simulink model "F4_CAN_Networking"  (R2018b)
settings: Solver=FixedStepAuto  StartTime=0.0  StopTime=10.0  FixedStep=0.25  RelTol=1e-3
undefined symbols (not defined in the file): CAN_MESSAGE
libraries: GPIO_Lib x9, CAN_Lib x7, STM32_Config_Lib x1, canmsglib x1
settings Model: Creator=reynaudp  LastModifiedBy=fenard1
settings SolverCC: InsertRTBMode=Always
settings DataIOCC: LimitDataPoints=on  SaveFormat=Array  ReturnWorkspaceOutputs=on
settings OptimizationCC: DefaultParameterBehavior=Inlined  DefaultUnderspecifiedDataType=single  InlineInvariantSignals=on  PassReuseOutputArgsAs=Individual arguments  LifeSpan=1
settings DebuggingCC: ReadBeforeWriteMsg=DisableAll  WriteAfterWriteMsg=DisableAll  WriteAfterReadMsg=DisableAll  SolverPrmCheckMsg=warning  MultiTaskDSMMsg=none  AllowSymbolicDim=off  StrictBusMsg=WarnOnBusTreatedAsVector  SFUnexpectedBacktrackingDiag=warning  SFNoUnconditionalDefaultTransitionDiag=warning  SFUndirectedBroadcastEventsDiag=error  SFExecutionAtInitializationDiag=none
settings HardwareCC: ProdBitPerPointer=32  ProdBitPerSizeT=32  ProdBitPerPtrDiffT=32  ProdLargestAtomicInteger=Integer  ProdWordSize=32  ProdHWDeviceType=STMicroelectronics->STM32 32-bit Cortex-M
settings ModelReferenceCC: UpdateModelReferenceTargets=IfOutOfDate  PropagateSignalLabelsOutOfModel=off
settings SFSimCC: SFSimEcho=off  SimUseLocalCustomCode=off  CompileTimeRecursionLimit=0  EnableRuntimeRecursion=off  MATLABDynamicMemAlloc=off
settings RTWCC: SystemTargetFile=stm32.tlc  TemplateMakefile=stm32.tmf  Description=stm32 (Embedded Target)  GenerateReport=on  RTWVerbose=off  RTWUseLocalCustomCode=off  Toolchain=Microsoft Windows SDK v7.1 | nmake (64-bit Windows)  IncludeHyperlinkInReport=on
settings CodeAppCC: IgnoreCustomStorageClasses=off  CustomSymbolStrType=$N$R$M  SimulinkBlockComments=off
settings STFCustomTargetCC: CodeReplacementLibrary=ARM CMSIS SIN COS  ParMdlRefBuildCompliant=on  IncludeMdlTerminateFcn=off  CombineOutputUpdateFcns=on  ERTCustomFileBanners=on  SupportContinuousTime=off  SupportNonInlinedSFcns=off  RemoveResetFunc=on  ParenthesesLevel=Maximum  CastingMode=Standards  MATLABClassNameForMDSCustomization=Simulink.SoftwareTarget.ERTCustomization  SystemTargetFile=stm32.tlc
settings ERTTargetCC: CodeReplacementLibrary=ARM CMSIS SIN COS  MultiwordLength=2048  CompOptLevelCompliant=off  ConcurrentExecutionCompliant=off  IncludeMdlTerminateFcn=off  ParenthesesLevel=Maximum  CastingMode=Standards  ModelStepFunctionPrototypeControlCompliant=off  CPPClassGenCompliant=off  UseToolchainInfoCompliant=off  ERTSrcFileBannerTemplate=sourceFileTemplate.cgt  ERTHdrFileBannerTemplate=sourceFileTemplate.cgt  ERTDataSrcFileTemplate=sourceFileTemplate.cgt  ERTDataHdrFileTemplate=sourceFileTemplate.cgt  ERTCustomFileTemplate=customRoutineProcess.tlc  ConvertIfToSwitch=off  SuppressUnreachableDefaultCases=off  EnableSignedLeftShifts=off  EnableSignedRightShifts=off
settings ConfigComp: CovMetricSettings=dw  CovHtmlReporting=on  CovSaveCumulativeToWorkspaceVar=on  CovSaveSingleToWorkspaceVar=on  CovExternalEMLEnable=off  CovSFcnEnable=off

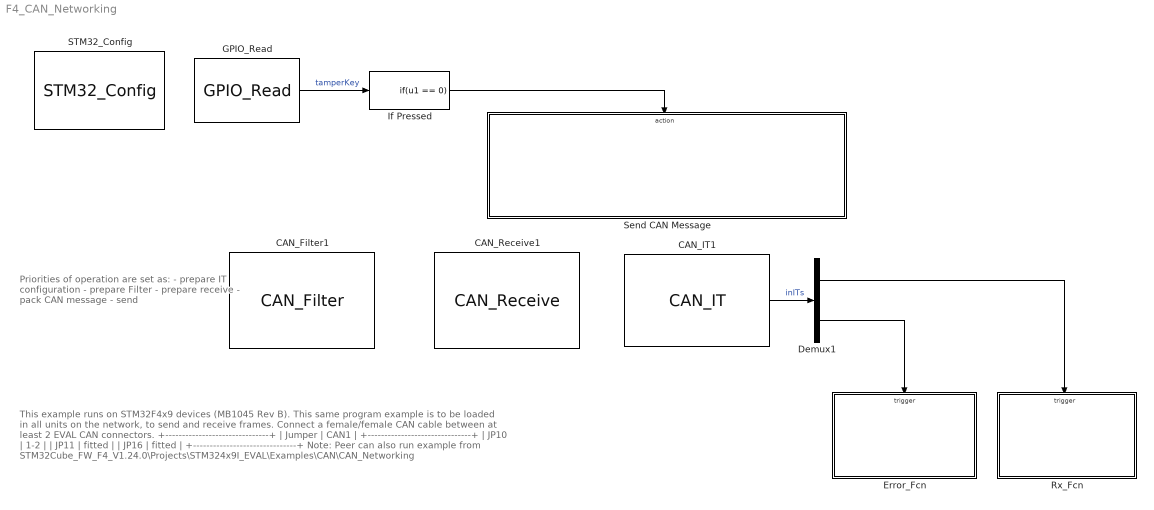
== system F4_CAN_Networking ==
  note: This example runs on STM32F4x9 devices (MB1045 Rev B).
      |
      | This same program example is to be loaded in all units on the network, to send and receive frames.
      |
      | Connect a female/female CAN cable between at least 2 EVAL CAN connectors.
      |
      | +-------------------------------+
      | | Jumper | CAN1 |
      | +-------------------------------+
      | | JP10 | 1-2 |
      | | JP11 | fitted |
      | | JP16 | fitted |
      | +-------------------------------+
      |
      | Note: Peer can also run example from STM32Cube_FW_F4_V1.24.0\Projects\STM324x9I_EVAL\Examples\CAN\CAN_Networking
  note: Priorities of operation are set as:
      | - prepare IT configuration
      | - prepare Filter
      | - prepare receive
      |
      | - pack CAN message
      | - send
  CAN_Filter1 : CAN_Lib/CAN_Filter  Priority=2  CAN_name=CAN1  CAN_Filter_Activation=on  CAN_Filter_Scale=CAN_FILTERSCALE_32BIT  CAN_Filter_Mask_Id_High=0  CAN_Filter_Mask_Id_Low=0  CAN_Filter_Id_High=0  CAN_Filter_Id_Low=0  CAN_Filter_FIFO_Assignment=CAN_FIFO0  CAN_Filter_Bank=0  CAN_Filter_Mode=CAN_FILTERMODE_IDMASK  CAN_Filter_Slave_Start_Bank=14
      settings: AttributesFormatString=Priority=%<Priority>  SourceProductName=Target Support Package - STM32 Adapter
  CAN_IT1 : CAN_Lib/CAN_IT  Priority=1  CAN_name=CAN1  CAN_Mode=Master  CAN_It=on  CAN_RX_It=on  CAN_TX_It=off  CAN_ERROR_It=on
      settings: AttributesFormatString=Priority=%<Priority>  SourceProductName=Target Support Package - STM32 Adapter
  CAN_Receive1 : CAN_Lib/CAN_Receive  Priority=3  CAN_name=CAN1  CAN_Mode=Master  CAN_It=on  CAN_Fifo=CAN_FIFO0
      settings: AttributesFormatString=Priority=%<Priority>  SourceProductName=Target Support Package - STM32 Adapter
  Demux1 : Demux  Outputs=2
  Error_Fcn : Subsystem  TreatAsAtomicUnit=on
  GPIO_Read : GPIO_Lib/GPIO_Read  Port_name=GPIOC  Pin_0=off  Pin_1=off  Pin_2=off  Pin_3=off  Pin_4=off  Pin_5=off  Pin_6=off  Pin_7=off  Pin_8=off  Pin_9=off  Pin_10=off  Pin_11=off  Pin_12=off  Pin_13=on  Pin_14=off  Pin_15=off  PinList=GPIOC13
      settings: SourceProductName=Target Support Package - STM32 Adapter
  If Pressed : If  IfExpression=u1 == 0  ShowElse=off
  Rx_Fcn : Subsystem  TreatAsAtomicUnit=on
  STM32_Config : STM32_Config_Lib/STM32_Config  Priority=0  Project_Path=.\  Config_File=F4_CAN_Networking.ioc  MCU_Name=STM32F439NIHx
      settings: SourceProductName=Target Support Package - STM32 Adapter
  Send CAN Message : Subsystem  TreatAsAtomicUnit=on  RTWFcnName=sendMessage
      settings: RTWFcnNameOpts=User specified
  wires:
  Demux1/2 -> Error_Fcn/Trigger
  CAN_IT1/1 -> Demux1/1  "inITs"
  Demux1/1 -> Rx_Fcn/Trigger
  GPIO_Read/1 -> If Pressed/1  "tamperKey"
  If Pressed/1 -> Send CAN Message/Action

== system F4_CAN_Networking/Error_Fcn ==
  Error_Fcn : TriggerPort  TriggerType=function-call  VariantControl=Variant
  CAN_Reset : CAN_Lib/CAN_Reset  CAN_name=CAN1
      settings: SourceProductName=Target Support Package - STM32 Adapter

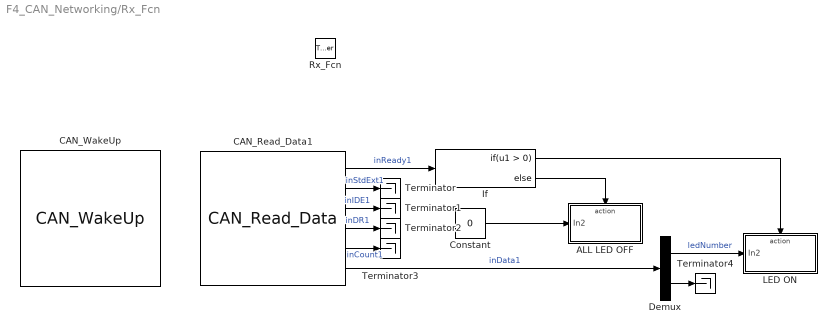
== system F4_CAN_Networking/Rx_Fcn ==
  Rx_Fcn : TriggerPort  TriggerType=function-call  VariantControl=Variant
  ALL LED OFF : Subsystem  TreatAsAtomicUnit=on
      settings: RTWSystemCode=Inline
  CAN_Read_Data1 : CAN_Lib/CAN_Read_Data  CAN_name=CAN1  CAN_Fifo=CAN_FIFO0  CAN_MsgType=off
      settings: SourceProductName=Target Support Package - STM32 Adapter
  CAN_WakeUp : CAN_Lib/CAN_WakeUp  CAN_name=CAN1  CAN_Mode=Master  CAN_It=on
      settings: SourceProductName=Target Support Package - STM32 Adapter
  Constant : Constant  Value=0  OutDataTypeStr=uint8
  Demux : Demux  Outputs=2
  If : If
  LED ON : Subsystem  TreatAsAtomicUnit=on
      settings: RTWSystemCode=Inline
  Terminator{,1..4} (5 alike) : Terminator
  wires:
  CAN_Read_Data1/6 -> Demux/1  "inData1"
  CAN_Read_Data1/1 -> If/1  "inReady1"
  If/1 -> LED ON/Action
  Demux/1 -> LED ON/1(In2)  "ledNumber"
  If/2 -> ALL LED OFF/Action
  Constant/1 -> ALL LED OFF/1(In2)
  CAN_Read_Data1/2 -> Terminator/1  "inStdExt1"
  CAN_Read_Data1/3 -> Terminator1/1  "inIDE1"
  CAN_Read_Data1/4 -> Terminator2/1  "inDR1"
  CAN_Read_Data1/5 -> Terminator3/1  "inCount1"
  Demux/2 -> Terminator4/1

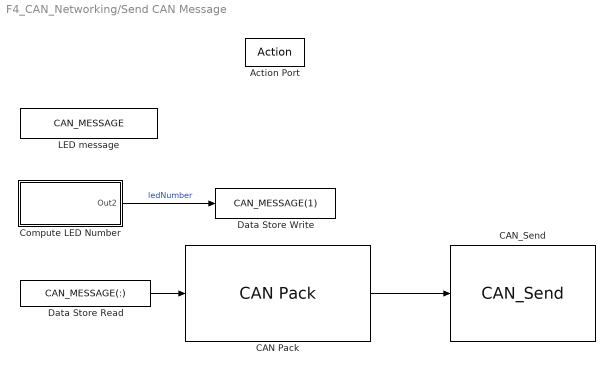
== system F4_CAN_Networking/Send CAN Message ==
  Action Port : ActionPort  ActionType=then
  CAN Pack : canmsglib/CAN Pack  Priority=22  MsgList=(none)  MsgName=CAN Msg  MsgIDType=Standard (11-bit identifier)  MsgIdentifier=801  MsgLength=2  SignalInfo=Signal1$0$8$1$1$1$0$1$0$-Inf$Inf$#  NSignals=1  StartBits=str2num('[int32(0)]')  SignalSizes=str2num('[int32(8)]')  ByteOrders=str2num('[int32(1)]')  DataTypes=str2num('[int32(1)]')  MultiplexTypes=str2num('[int32(1)]')  MultiplexValues=str2num('[double(0)]')  Factors=str2num('[double(1)]')  Offsets=str2num('[double(0)]')  Minimums=str2num('[double(-Inf)]')  Maximums=str2num('[double(Inf)]')  Remote=off  ApplyMinMax=off  BusOutput=off
      settings: AttributesFormatString=Priority=%<Priority>  SourceProductName=Simulink Real-Time  SourceProductBaseCode=XP  DataFormat=raw data
  CAN_Send : CAN_Lib/CAN_Send  Priority=23  CAN_name=CAN1  CAN_Mode=Master  CAN_It=off  CAN_MsgType=on
      settings: AttributesFormatString=Priority=%<Priority>  SourceProductName=Target Support Package - STM32 Adapter
  Compute LED Number : Subsystem  Priority=21  TreatAsAtomicUnit=on  RTWFcnName=computeLedNumber
      settings: AttributesFormatString=Priority=%<Priority>  RTWFcnNameOpts=User specified
  Data Store Read : DataStoreRead  DataStoreName=CAN_MESSAGE  DataStoreElements=CAN_MESSAGE(:)
  Data Store Write : DataStoreWrite  DataStoreName=CAN_MESSAGE  DataStoreElements=CAN_MESSAGE(1)
  LED message : DataStoreMemory  DataStoreName=CAN_MESSAGE  ReadBeforeWriteMsg=warning  WriteAfterWriteMsg=warning  WriteAfterReadMsg=warning  InitialValue=[1, 173]  ShowAdditionalParam=off  OutDataTypeStr=uint8
  wires:
  Compute LED Number/1(Out2) -> Data Store Write/1  "ledNumber"
  CAN Pack/1 -> CAN_Send/1
  Data Store Read/1 -> CAN Pack/1

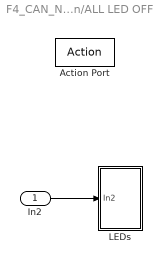
== system F4_CAN_Networking/Rx_Fcn/ALL LED OFF ==
  In2 : Inport  OutDataTypeStr=uint8
  Action Port : ActionPort  ActionType=else
  LEDs : Subsystem
  wires:
  In2/1 -> LEDs/1(In2)

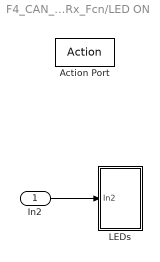
== system F4_CAN_Networking/Rx_Fcn/LED ON ==
  In2 : Inport  OutDataTypeStr=uint8
  Action Port : ActionPort  ActionType=then
  LEDs : Subsystem  TreatAsAtomicUnit=on  RTWFcnName=setLed
      settings: RTWFcnNameOpts=User specified
  wires:
  In2/1 -> LEDs/1(In2)

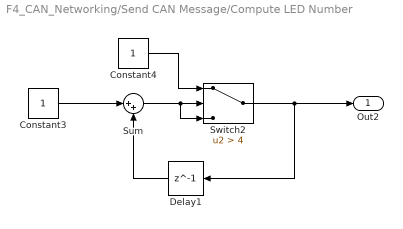
== system F4_CAN_Networking/Send CAN Message/Compute LED Number ==
  Constant3 : Constant  OutDataTypeStr=uint8
  Constant4 : Constant  OutDataTypeStr=uint8
  Delay1 : Delay  DelayLength=1  InitialCondition=0
  Sum : Sum  Inputs=|++
  Switch2 : Switch  Criteria=u2 > Threshold  Threshold=4  OutDataTypeStr=uint8
  Out2 : Outport
  wires:
  Sum/1 -> Switch2/3, Switch2/2
  Constant4/1 -> Switch2/1
  Delay1/1 -> Sum/2
  Constant3/1 -> Sum/1
  Switch2/1 -> Delay1/1, Out2/1

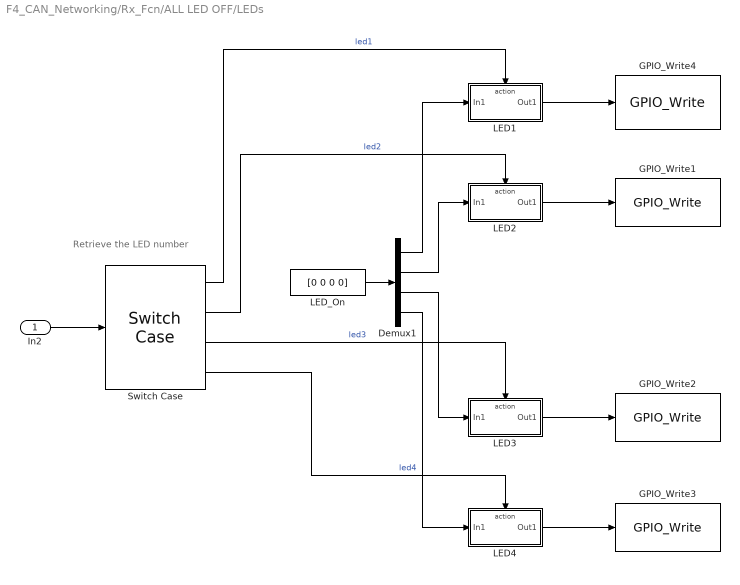
== system F4_CAN_Networking/Rx_Fcn/ALL LED OFF/LEDs ==
  note: Retrieve the LED number
  In2 : Inport  OutDataTypeStr=uint8
  Demux1 : Demux
  GPIO_Write1 : GPIO_Lib/GPIO_Write  Port_name=GPIOG  Pin0=off  Toggle_Pin0=off  Pin1=off  Toggle_Pin1=off  Pin2=off  Toggle_Pin2=off  Pin3=off  Toggle_Pin3=off  Pin4=off  Toggle_Pin4=off  Pin5=off  Toggle_Pin5=off  Pin6=off  Toggle_Pin6=off  Pin7=on  Toggle_Pin7=off  Pin8=off  Toggle_Pin8=off  Pin9=off  Toggle_Pin9=off  Pin10=off  Toggle_Pin10=off  Pin11=off  Toggle_Pin11=off  Pin12=off  Toggle_Pin12=off  Pin13=off  Toggle_Pin13=off  Pin14=off  Toggle_Pin14=off  Pin15=off  Toggle_Pin15=off  PinList="GPIOG6   7  10  12"
      settings: SourceProductName=Target Support Package - STM32 Adapter
  GPIO_Write2 : GPIO_Lib/GPIO_Write  Port_name=GPIOG  Pin0=off  Toggle_Pin0=off  Pin1=off  Toggle_Pin1=off  Pin2=off  Toggle_Pin2=off  Pin3=off  Toggle_Pin3=off  Pin4=off  Toggle_Pin4=off  Pin5=off  Toggle_Pin5=off  Pin6=off  Toggle_Pin6=off  Pin7=off  Toggle_Pin7=off  Pin8=off  Toggle_Pin8=off  Pin9=off  Toggle_Pin9=off  Pin10=on  Toggle_Pin10=off  Pin11=off  Toggle_Pin11=off  Pin12=off  Toggle_Pin12=off  Pin13=off  Toggle_Pin13=off  Pin14=off  Toggle_Pin14=off  Pin15=off  Toggle_Pin15=off  PinList="GPIOG6   7  10  12"
      settings: SourceProductName=Target Support Package - STM32 Adapter
  GPIO_Write3 : GPIO_Lib/GPIO_Write  Port_name=GPIOG  Pin0=off  Toggle_Pin0=off  Pin1=off  Toggle_Pin1=off  Pin2=off  Toggle_Pin2=off  Pin3=off  Toggle_Pin3=off  Pin4=off  Toggle_Pin4=off  Pin5=off  Toggle_Pin5=off  Pin6=off  Toggle_Pin6=off  Pin7=off  Toggle_Pin7=off  Pin8=off  Toggle_Pin8=off  Pin9=off  Toggle_Pin9=off  Pin10=off  Toggle_Pin10=off  Pin11=off  Toggle_Pin11=off  Pin12=on  Toggle_Pin12=off  Pin13=off  Toggle_Pin13=off  Pin14=off  Toggle_Pin14=off  Pin15=off  Toggle_Pin15=off  PinList="GPIOG6   7  10  12"
      settings: SourceProductName=Target Support Package - STM32 Adapter
  GPIO_Write4 : GPIO_Lib/GPIO_Write  Port_name=GPIOG  Pin0=off  Toggle_Pin0=off  Pin1=off  Toggle_Pin1=off  Pin2=off  Toggle_Pin2=off  Pin3=off  Toggle_Pin3=off  Pin4=off  Toggle_Pin4=off  Pin5=off  Toggle_Pin5=off  Pin6=on  Toggle_Pin6=off  Pin7=off  Toggle_Pin7=off  Pin8=off  Toggle_Pin8=off  Pin9=off  Toggle_Pin9=off  Pin10=off  Toggle_Pin10=off  Pin11=off  Toggle_Pin11=off  Pin12=off  Toggle_Pin12=off  Pin13=off  Toggle_Pin13=off  Pin14=off  Toggle_Pin14=off  Pin15=off  Toggle_Pin15=off  PinList="GPIOG6   7  10  12"
      settings: SourceProductName=Target Support Package - STM32 Adapter
  LED1 : Subsystem  TreatAsAtomicUnit=on
  LED2 : Subsystem  TreatAsAtomicUnit=on
  LED3 : Subsystem  TreatAsAtomicUnit=on
  LED4 : Subsystem  TreatAsAtomicUnit=on
  LED_On : Constant  Value=[0 0 0 0]  OutDataTypeStr=uint32
  Switch Case : SwitchCase  CaseConditions={1,2,3,4}  ShowDefaultCase=off
  wires:
  Demux1/2 -> LED2/1(In1)
  LED_On/1 -> Demux1/1
  Switch Case/3 -> LED3/Action  "led3"
  Demux1/3 -> LED3/1(In1)
  LED4/1(Out1) -> GPIO_Write3/1
  LED1/1(Out1) -> GPIO_Write4/1
  In2/1 -> Switch Case/1
  LED3/1(Out1) -> GPIO_Write2/1
  Switch Case/4 -> LED4/Action  "led4"
  Demux1/4 -> LED4/1(In1)
  LED2/1(Out1) -> GPIO_Write1/1
  Switch Case/1 -> LED1/Action  "led1"
  Switch Case/2 -> LED2/Action  "led2"
  Demux1/1 -> LED1/1(In1)

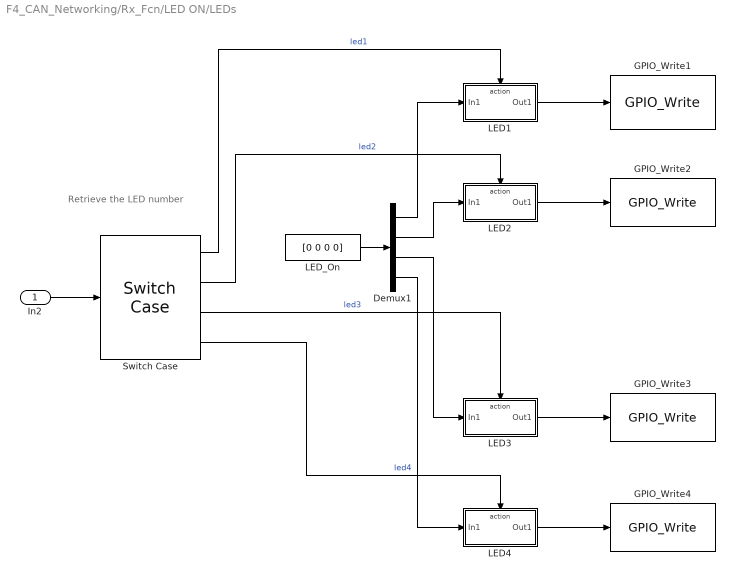
== system F4_CAN_Networking/Rx_Fcn/LED ON/LEDs ==
  note: Retrieve the LED number
  In2 : Inport  OutDataTypeStr=uint8
  Demux1 : Demux
  GPIO_Write1 : GPIO_Lib/GPIO_Write  Port_name=GPIOG  Pin0=off  Toggle_Pin0=off  Pin1=off  Toggle_Pin1=off  Pin2=off  Toggle_Pin2=off  Pin3=off  Toggle_Pin3=off  Pin4=off  Toggle_Pin4=off  Pin5=off  Toggle_Pin5=off  Pin6=on  Toggle_Pin6=off  Pin7=off  Toggle_Pin7=off  Pin8=off  Toggle_Pin8=off  Pin9=off  Toggle_Pin9=off  Pin10=off  Toggle_Pin10=off  Pin11=off  Toggle_Pin11=off  Pin12=off  Toggle_Pin12=off  Pin13=off  Toggle_Pin13=off  Pin14=off  Toggle_Pin14=off  Pin15=off  Toggle_Pin15=off  PinList="GPIOG6   7  10  12"
      settings: SourceProductName=Target Support Package - STM32 Adapter
  GPIO_Write2 : GPIO_Lib/GPIO_Write  Port_name=GPIOG  Pin0=off  Toggle_Pin0=off  Pin1=off  Toggle_Pin1=off  Pin2=off  Toggle_Pin2=off  Pin3=off  Toggle_Pin3=off  Pin4=off  Toggle_Pin4=off  Pin5=off  Toggle_Pin5=off  Pin6=off  Toggle_Pin6=off  Pin7=on  Toggle_Pin7=off  Pin8=off  Toggle_Pin8=off  Pin9=off  Toggle_Pin9=off  Pin10=off  Toggle_Pin10=off  Pin11=off  Toggle_Pin11=off  Pin12=off  Toggle_Pin12=off  Pin13=off  Toggle_Pin13=off  Pin14=off  Toggle_Pin14=off  Pin15=off  Toggle_Pin15=off  PinList="GPIOG6   7  10  12"
      settings: SourceProductName=Target Support Package - STM32 Adapter
  GPIO_Write3 : GPIO_Lib/GPIO_Write  Port_name=GPIOG  Pin0=off  Toggle_Pin0=off  Pin1=off  Toggle_Pin1=off  Pin2=off  Toggle_Pin2=off  Pin3=off  Toggle_Pin3=off  Pin4=off  Toggle_Pin4=off  Pin5=off  Toggle_Pin5=off  Pin6=off  Toggle_Pin6=off  Pin7=off  Toggle_Pin7=off  Pin8=off  Toggle_Pin8=off  Pin9=off  Toggle_Pin9=off  Pin10=on  Toggle_Pin10=off  Pin11=off  Toggle_Pin11=off  Pin12=off  Toggle_Pin12=off  Pin13=off  Toggle_Pin13=off  Pin14=off  Toggle_Pin14=off  Pin15=off  Toggle_Pin15=off  PinList="GPIOG6   7  10  12"
      settings: SourceProductName=Target Support Package - STM32 Adapter
  GPIO_Write4 : GPIO_Lib/GPIO_Write  Port_name=GPIOG  Pin0=off  Toggle_Pin0=off  Pin1=off  Toggle_Pin1=off  Pin2=off  Toggle_Pin2=off  Pin3=off  Toggle_Pin3=off  Pin4=off  Toggle_Pin4=off  Pin5=off  Toggle_Pin5=off  Pin6=off  Toggle_Pin6=off  Pin7=off  Toggle_Pin7=off  Pin8=off  Toggle_Pin8=off  Pin9=off  Toggle_Pin9=off  Pin10=off  Toggle_Pin10=off  Pin11=off  Toggle_Pin11=off  Pin12=on  Toggle_Pin12=off  Pin13=off  Toggle_Pin13=off  Pin14=off  Toggle_Pin14=off  Pin15=off  Toggle_Pin15=off  PinList="GPIOG6   7  10  12"
      settings: SourceProductName=Target Support Package - STM32 Adapter
  LED1 : Subsystem  TreatAsAtomicUnit=on
  LED2 : Subsystem  TreatAsAtomicUnit=on
  LED3 : Subsystem  TreatAsAtomicUnit=on
  LED4 : Subsystem  TreatAsAtomicUnit=on
  LED_On : Constant  Value=[0 0 0 0]  OutDataTypeStr=uint32
  Switch Case : SwitchCase  CaseConditions={1,2,3,4}  ShowDefaultCase=off
  wires:
  Demux1/2 -> LED2/1(In1)
  LED_On/1 -> Demux1/1
  Switch Case/3 -> LED3/Action  "led3"
  Demux1/3 -> LED3/1(In1)
  LED4/1(Out1) -> GPIO_Write4/1
  LED1/1(Out1) -> GPIO_Write1/1
  In2/1 -> Switch Case/1
  LED3/1(Out1) -> GPIO_Write3/1
  Switch Case/4 -> LED4/Action  "led4"
  Demux1/4 -> LED4/1(In1)
  LED2/1(Out1) -> GPIO_Write2/1
  Switch Case/1 -> LED1/Action  "led1"
  Switch Case/2 -> LED2/Action  "led2"
  Demux1/1 -> LED1/1(In1)

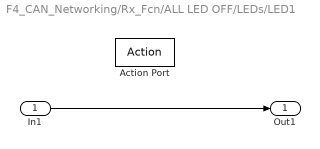
== system F4_CAN_Networking/Rx_Fcn/ALL LED OFF/LEDs/LED1 ==
  In1 : Inport  OutDataTypeStr=uint32
  Action Port : ActionPort  ActionType=case
  Out1 : Outport  OutDataTypeStr=uint32  OutputWhenDisabled=reset  InitialOutput=[1]
  wires:
  In1/1 -> Out1/1

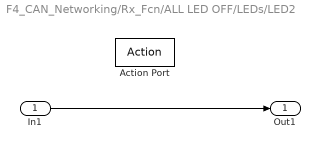
== system F4_CAN_Networking/Rx_Fcn/ALL LED OFF/LEDs/LED2 ==
  In1 : Inport
  Action Port : ActionPort  ActionType=case
  Out1 : Outport  OutDataTypeStr=uint32  OutputWhenDisabled=reset  InitialOutput=[1]
  wires:
  In1/1 -> Out1/1

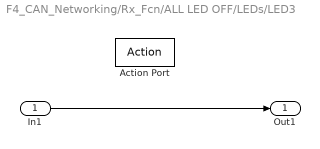
== system F4_CAN_Networking/Rx_Fcn/ALL LED OFF/LEDs/LED3 ==
  In1 : Inport
  Action Port : ActionPort  ActionType=case
  Out1 : Outport  OutputWhenDisabled=reset  InitialOutput=[1]
  wires:
  In1/1 -> Out1/1

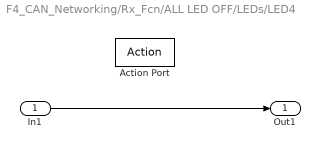
== system F4_CAN_Networking/Rx_Fcn/ALL LED OFF/LEDs/LED4 ==
  In1 : Inport
  Action Port : ActionPort  ActionType=case
  Out1 : Outport  OutputWhenDisabled=reset  InitialOutput=[1]
  wires:
  In1/1 -> Out1/1

== system F4_CAN_Networking/Rx_Fcn/LED ON/LEDs/LED1 ==
  In1 : Inport  OutDataTypeStr=uint32
  Action Port : ActionPort  ActionType=case
  Out1 : Outport  OutDataTypeStr=uint32  OutputWhenDisabled=reset  InitialOutput=[1]
  wires:
  In1/1 -> Out1/1

== system F4_CAN_Networking/Rx_Fcn/LED ON/LEDs/LED2 ==
  In1 : Inport
  Action Port : ActionPort  ActionType=case
  Out1 : Outport  OutDataTypeStr=uint32  OutputWhenDisabled=reset  InitialOutput=[1]
  wires:
  In1/1 -> Out1/1

== system F4_CAN_Networking/Rx_Fcn/LED ON/LEDs/LED3 ==
  In1 : Inport
  Action Port : ActionPort  ActionType=case
  Out1 : Outport  OutputWhenDisabled=reset  InitialOutput=[1]
  wires:
  In1/1 -> Out1/1

== system F4_CAN_Networking/Rx_Fcn/LED ON/LEDs/LED4 ==
  In1 : Inport
  Action Port : ActionPort  ActionType=case
  Out1 : Outport  OutputWhenDisabled=reset  InitialOutput=[1]
  wires:
  In1/1 -> Out1/1
